simulink model "Mass_Spring_Damper"  (R2025b)
settings: Solver=VariableStepAuto  StartTime=0.0  StopTime=30.0  MaxStep=0.001  RelTol=1e-3
settings Model: Creator=user  LastModifiedBy=user

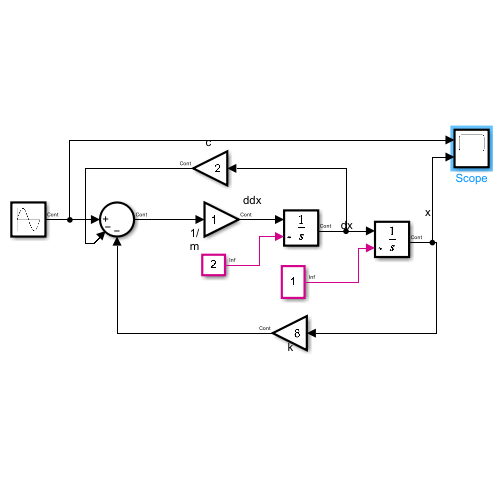
[thumbnail: Simulink's stored preview of the top-level diagram]
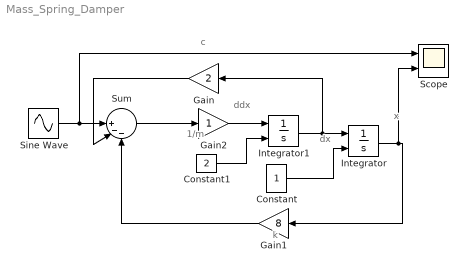
== system Mass_Spring_Damper ==
  note: 1/m
  note: c
  note: k
  note: ddx
  note: x
  note: dx
  Constant : Constant
  Constant1 : Constant  Value=2
  Gain : Gain  Gain=2
  Gain1 : Gain  Gain=8
  Gain2 : Gain
  Integrator : Integrator  InitialConditionSource=external  InitialCondition=1
  Integrator1 : Integrator  InitialConditionSource=external  InitialCondition=2
  Scope : Scope  NumInputPorts=2
      settings: ActiveDisplayYMinimum=-0.54878434004040855  ActiveDisplayYMaximum=1.3726423405460797
  Sine Wave : Sin  Amplitude=2  Frequency=2  SampleTime=0
  Sum : Sum  Inputs=||+--
  wires:
  Constant/1 -> Integrator/2
  Constant1/1 -> Integrator1/2
  Sine Wave/1 -> Scope/1, Sum/1
  Sum/1 -> Gain2/1
  Gain1/1 -> Sum/3
  Gain2/1 -> Integrator1/1
  Gain/1 -> Sum/2
  Integrator1/1 -> Gain/1, Integrator/1
  Integrator/1 -> Gain1/1, Scope/2
